simulink model "EV_thermal_charger_2015a_jmaab"  (R2015a)
settings: Solver=ode3  StartTime=0.0  StopTime=1800  FixedStep=sampling_time  RelTol=1e-3
PreLoadFcn:
  | run('init_setting.m')
PostLoadFcn:
  | %set_param(gcs, 'SimulationCommand', 'update');
  | %load('save_param/save_P_Charger', 'P_Charger');
  | %load('save_param/save_T_User_set_temp_degC','T_User_set_temp_degC');
  | %load('save_param/save_ENV_PNT_PTTH_Temp_add_degC','ENV_PNT_PTTH_Temp_add_degC');
  | %load('save_param/save_ENV_PNT_CABIN_Temp_add_degC','ENV_PNT_CABIN_Temp_add_degC');
  | %load('save_param/save_ENV_PNT_PHI_Sunlight_W','ENV_PNT_PHI_Sunlight_W');
  | %load('save_param/save_ENV_PNT_Outside_Temp_ini_degC','ENV_PNT_Outside_Temp_ini_degC');
undefined symbols (not defined in the file or in its folder): BK_PNT_Pow_UL, BK_PNT_ReGene_vel_limit_DN_kmph, BK_PNT_ReGene_vel_limit_UP_kmph, BK_PNT_Tau_brake, Brk_LL, Brk_PGain, Brk_UL, BT_PNT_Hi_C_pol_hi_batt, BT_PNT_Hi_Capa_hi_batt_F, BT_PNT_Hi_ocv_SOC_hi_batt_OCV_V_table, BT_PNT_Hi_ocv_SOC_hi_batt_OCV_V_table_x_SOC, BT_PNT_Hi_R_hi_batt_cell, BT_PNT_Hi_R_pol_hi_batt, BT_PNT_Hi_SOC_MAX_hi_batt, BT_PNT_Hi_SOC_MIN_hi_batt, BT_PNT_Hi_SOC_START_hi_batt, BT_PNT_Lo_Capa_lo_batt_F, BT_PNT_Lo_ocv_SOC_lo_batt_OCV_V_table, BT_PNT_Lo_ocv_SOC_lo_batt_OCV_V_table_x_SOC, BT_PNT_Lo_R_lo_batt_ohm, BT_PNT_Lo_SOC_MAX_lo_batt, BT_PNT_Lo_SOC_MIN_lo_batt, BT_PNT_Lo_SOC_START_lo_batt, BTTH_CNT_P_BT_Heater_W, BTTH_CNT_P_BT_Heater_W_x_BTCells_degC, BTTH_CNT_Voltage_BTFan_V, BTTH_CNT_Voltage_BTFan_V_x_BTCells_degC, BTTH_PNT_BT_Heat_Resi_KpW, BTTH_PNT_BT_Heat_Resi_KpW_x_Wind_m3ps, BTTH_PNT_BT_Heater2BTCells_Heat_Resi_KpW, BTTH_PNT_BT_Heater_Heat_Capa_JpK, BTTH_PNT_BTBlock2BTAir_Heat_Resi_KpW, BTTH_PNT_BTBlock_Heat_Capa_JpK, BTTH_PNT_BTCells2BTBlock_Heat_Resi_KpW, BTTH_PNT_BTCells_Heat_Capa_JpK, BTTH_PNT_v_BTFan_Wind_vel_mps, BTTH_PNT_v_BTFan_Wind_vel_mps_x_V_BTFan, CATH_CNT_P_Aircon_W_LL, CATH_CNT_P_Aircon_W_UL, CATH_CNT_P_Gain_Aircon, CATH_CNT_P_Gain_PTC_Heater, CATH_CNT_P_Gain_SeatHT, CATH_CNT_P_PTC_Heater, CATH_CNT_P_PTC_Heater_W_LL, CATH_CNT_P_PTC_Heater_W_UL, CATH_CNT_P_PTC_Heater_x_T_Outside_temp_degC, CATH_CNT_P_SeatHT_W_LL, CATH_CNT_P_SeatHT_W_UL, CATH_CNT_PGain_Temp_blowout, CATH_CNT_T_Aircon_Indoor_degC, CATH_CNT_T_Aircon_Indoor_degC_x_T_blowout_degC, CATH_CNT_T_PTC_Heater_degC_UL, CATH_CNT_T_SeatHT_Temp_degC, CATH_CNT_T_SeatHT_Temp_degC_x_T_blowout_degC, CATH_CNT_V_HVAC_Fan, CATH_CNT_V_HVAC_Fan_x_T_blowout_degC, CATH_CNT_V_RDFan_V, CATH_CNT_V_RDFan_x_P_Aircon_W, CATH_PNT_Air_Convection_Heat_Resi_KpW, CATH_PNT_Air_Convection_Heat_Resi_x_mps ... (+142)
undefined symbols (not defined in the file): ACC_D_Gain, ACC_I_Gain, ACC_P_Gain
libraries: METI_Lib_vehicle_model x52, simulink x35
(part 1 of 6)
PreSaveFcn:
  | %save('save_param/save_P_Charger', 'P_Charger');
  | %save('save_param/save_T_User_set_temp_degC', 'T_User_set_temp_degC');
  | %save('save_param/save_ENV_PNT_PTTH_Temp_add_degC', 'ENV_PNT_PTTH_Temp_add_degC');
  | %save('save_param/save_ENV_PNT_CABIN_Temp_add_degC', 'ENV_PNT_CABIN_Temp_add_degC');
  | %save('save_param/save_ENV_PNT_PHI_Sunlight_W', 'ENV_PNT_PHI_Sunlight_W');
  | %save('save_param/save_ENV_PNT_Outside_Temp_ini_degC', 'ENV_PNT_Outside_Temp_ini_degC');
settings Model: Creator=AZAPA  LastModifiedBy=E00026
settings OptimizationCC: EfficientMapNaN2IntZero=off
settings DebuggingCC: SFInvalidInputDataAccessInChartInitDiag=none  SFNoUnconditionalDefaultTransitionDiag=none
settings HardwareCC: TargetBitPerPointer=64  TargetLongLongMode=on  TargetIntDivRoundTo=Zero  TargetEndianess=LittleEndian  TargetWordSize=64  TargetHWDeviceType=MATLAB Host  ProdEqTarget=off
settings CodeAppCC: MaxIdLength=128
settings GRTTargetCC: CombineOutputUpdateFcns=off  GRTInterface=on

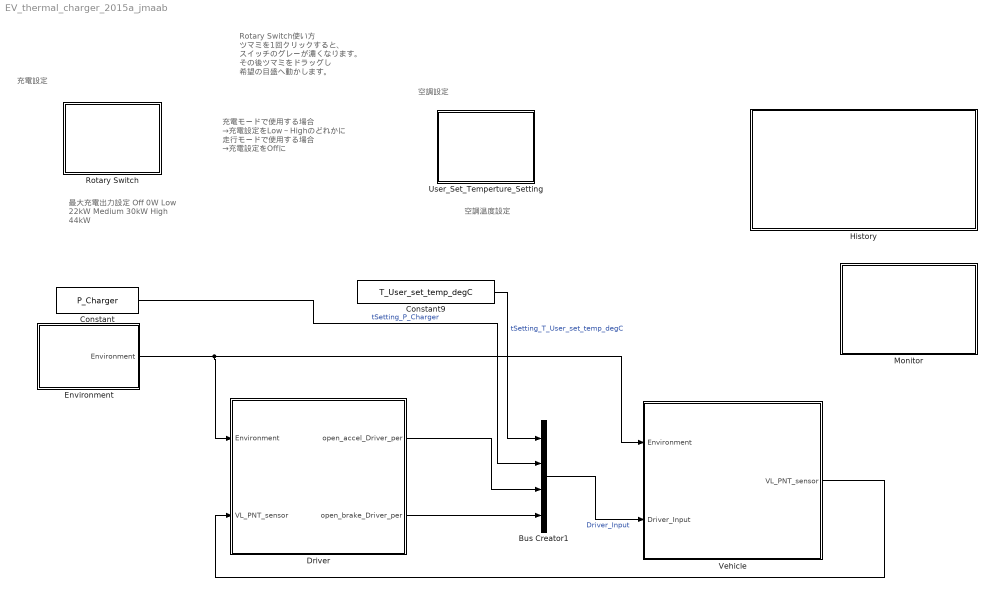
== system EV_thermal_charger_2015a_jmaab ==
  note: 充電モードで使用する場合
      | →充電設定をLow～Highのどれかに
      |
      | 走行モードで使用する場合
      | →充電設定をOffに
  note: 充電設定
  note: 空調温度設定
  note: 空調設定
  note: 最大充電出力設定
      | Off 0W
      | Low 22kW
      | Medium 30kW
      | High 44kW
  note: Rotary Switch使い方
      | ツマミを1回クリックすると、
      | スイッチのグレーが濃くなります。
      | その後ツマミをドラッグし
      | 希望の目盛へ動かします。
  Bus Creator1 : BusCreator  Inputs=4
  Constant : Constant  Value=P_Charger
  Constant9 : Constant  Value=T_User_set_temp_degC
  Driver : Subsystem
      mask Display: image(imread('picture\ドライバ.png'))
  Environment : Subsystem
  History : Subsystem
  Monitor : Subsystem
  Rotary Switch : Subsystem  DialogController=hmiCreateDDGDialog  IsWebBlock=on  mask(MathWorksWebBlock){webBlockId=88c50587-98df-4da6-abec-7a3537762cf8, webBlockType=discreteknob, ShowInLibBrowser=on, ShowInitialText=on, HMISrcModelName=tpeaf5fb4a_b3bf_4f70_b0c1_9b4aa428c6f5}
      mask prompts: webBlockId "WebBlock Id"; webBlockType "WebBlock Type"; HMISrcModelName "Source Model"
      mask help: 値を設定してパラメーターまたは変数を調整します。
      mask Help: helpview([docroot '/mapfiles/simulink.map'], 'hmi_rotary_switch')
      mask Display:
      | if strcmp(get_param(bdroot(gcb),'BlockDiagramType'),'library')
      |  image([(matlabroot) '/toolbox/simulink/hmi/icons/DiscreteKnob.png'])
      | end
  User_Set_Temperture_Setting : Subsystem  DialogController=hmiCreateDDGDialog  IsWebBlock=on  mask(MathWorksWebBlock){webBlockId=37ee7956-8de0-466d-b842-934e6700f2c4, webBlockType=discreteknob, ShowInLibBrowser=on, ShowInitialText=on, HMISrcModelName=tpeaf5fb4a_b3bf_4f70_b0c1_9b4aa428c6f5}
      mask prompts: webBlockId "WebBlock Id"; webBlockType "WebBlock Type"; HMISrcModelName "Source Model"
      mask help: 値を設定してパラメーターまたは変数を調整します。
      mask Help: helpview([docroot '/mapfiles/simulink.map'], 'hmi_rotary_switch')
      mask Display:
      | if strcmp(get_param(bdroot(gcb),'BlockDiagramType'),'library')
      |  image([(matlabroot) '/toolbox/simulink/hmi/icons/DiscreteKnob.png'])
      | end
  Vehicle : Subsystem
      mask Display: image(imread('picture\電気負荷.png'))
  wires:
  Vehicle/1(VL_PNT_sensor) -> Driver/2(VL_PNT_sensor)
  Driver/1(open_accel_Driver_per) -> Bus Creator1/3
  Driver/2(open_brake_Driver_per) -> Bus Creator1/4
  Constant/1 -> Bus Creator1/2  "tSetting_P_Charger"
  Constant9/1 -> Bus Creator1/1  "tSetting_T_User_set_temp_degC"
  Environment/1(Environment) -> Driver/1(Environment), Vehicle/1(Environment)
  Bus Creator1/1 -> Vehicle/2(Driver_Input)  "Driver_Input"

== system EV_thermal_charger_2015a_jmaab/Driver ==
  Environment : Inport
  VL_PNT_sensor : Inport  Port=2
  Bus Selector : BusSelector  OutputSignals=tgt_v_kmph
  Bus Selector1 : BusSelector  OutputSignals=v_VL_PNT_kmph
  Caliculate_Driving_State : Subsystem
  Caliculate_Opeining_Accel : Subsystem
  Caliculate_Opening_Brake : Subsystem
  Memory2 : Memory  InheritSampleTime=on
  open_accel_Driver_per : Outport
  open_brake_Driver_per : Outport  Port=2
  tag scope: tScope_accel=global, tScope_brake=global, tScope_v_Vehicle=global, tScope_v_tgt=global
  wires:
  Memory2/1 -> [tScope_v_Vehicle], Caliculate_Opening_Brake/1(v_VL_PNT_kmph), Caliculate_Opeining_Accel/1(v_VL_PNT_kmph)
  Caliculate_Opeining_Accel/1(open_accel_Driver_per) -> open_accel_Driver_per/1, [tScope_accel], Caliculate_Opening_Brake/3(open_accel_Driver_per)
  Caliculate_Opening_Brake/1(open_brake_Driver_per) -> open_brake_Driver_per/1, [tScope_brake], Caliculate_Driving_State/1(open_brake_Driver_per)
  VL_PNT_sensor/1 -> Bus Selector1/1
  Environment/1 -> Bus Selector/1
  Bus Selector/1 -> Caliculate_Driving_State/2(tgt_v_kmph), Caliculate_Opening_Brake/2(tgt_v_kmph), Caliculate_Opeining_Accel/2(tgt_v_kmph), [tScope_v_tgt]  "<tgt_v_kmph>"
  Bus Selector1/1 -> Memory2/1  "<v_VL_PNT_kmph>"

== system EV_thermal_charger_2015a_jmaab/Environment ==
  note: 車外気温設定
      | VeryCold -30℃
      | Cold 0℃
      | Warm 20℃
      | VeryHot 40℃
  note: 気象設定（直射日光の有無）
      | Night 日射熱量 0W
      | Cloudy 日射熱量 100W
      | Sunny 日射熱量 1000W
  note: 気象条件設定
  note: Rotary Switch使い方
      | ツマミを1回クリックすると、
      | スイッチのグレーが濃くなります。
      | その後ツマミをドラッグし
      | 希望の目盛へ動かします。
  note: スタート時
      | 車室温度設定
      | 直射日光下で駐車した状態では
      | 車室温度は外気温より高くなる
  note: スタート時パワトレ・パワエレ
      | HOT/COLD設定
      | COLD 外気温と同じ温度から
      | HOT 外気温+40℃から
  note: 車両条件設定
  note: 充電モードでは走行しないので
      | 目標車速を0にする
  Bus Creator2 : BusCreator  Inputs=5
  CABIN_Temp_add : Subsystem  DialogController=hmiCreateDDGDialog  IsWebBlock=on  mask(MathWorksWebBlock){webBlockId=d4d8367f-57c7-4656-8fe5-c97b2c29613b, webBlockType=discreteknob, ShowInLibBrowser=on, ShowInitialText=on, HMISrcModelName=tpeaf5fb4a_b3bf_4f70_b0c1_9b4aa428c6f5}
      mask prompts: webBlockId "WebBlock Id"; webBlockType "WebBlock Type"; HMISrcModelName "Source Model"
      mask help: 値を設定してパラメーターまたは変数を調整します。
      mask Help: helpview([docroot '/mapfiles/simulink.map'], 'hmi_rotary_switch')
      mask Display:
      | if strcmp(get_param(bdroot(gcb),'BlockDiagramType'),'library')
      |  image([(matlabroot) '/toolbox/simulink/hmi/icons/DiscreteKnob.png'])
      | end
  COLD/HOT : Subsystem  DialogController=hmiCreateDDGDialog  IsWebBlock=on  mask(MathWorksWebBlock){webBlockId=ec53c6ff-a8cf-4237-bb99-052eb2fa9088, webBlockType=discreteknob, ShowInLibBrowser=on, ShowInitialText=on, HMISrcModelName=tpeaf5fb4a_b3bf_4f70_b0c1_9b4aa428c6f5}
      mask prompts: webBlockId "WebBlock Id"; webBlockType "WebBlock Type"; HMISrcModelName "Source Model"
      mask help: 値を設定してパラメーターまたは変数を調整します。
      mask Help: helpview([docroot '/mapfiles/simulink.map'], 'hmi_rotary_switch')
      mask Display:
      | if strcmp(get_param(bdroot(gcb),'BlockDiagramType'),'library')
      |  image([(matlabroot) '/toolbox/simulink/hmi/icons/DiscreteKnob.png'])
      | end
  Constant3 : Constant  Value=P_Charger
  Constant4 : Constant  Value=0
  Constant5 : Constant  Value=ENV_PNT_PTTH_Temp_add_degC
  Constant6 : Constant  Value=ENV_PNT_CABIN_Temp_add_degC
  Constant7 : Constant  Value=ENV_PNT_PHI_Sunlight_W
  Constant8 : Constant  Value=ENV_PNT_Outside_Temp_ini_degC
  From Workspace : FromWorkspace  VariableName=jc08  SampleTime=0
  From Workspace2 : FromWorkspace  VariableName=wltc_class3b  SampleTime=0
  Manual Switch2 : ManualSwitch  CurrentSetting=0
  Outside_Temperture_Setting : Subsystem  DialogController=hmiCreateDDGDialog  IsWebBlock=on  mask(MathWorksWebBlock){webBlockId=d913990a-62c7-4b41-8bbd-c48c7457c0a7, webBlockType=discreteknob, ShowInLibBrowser=on, ShowInitialText=on, HMISrcModelName=tpeaf5fb4a_b3bf_4f70_b0c1_9b4aa428c6f5}
      mask prompts: webBlockId "WebBlock Id"; webBlockType "WebBlock Type"; HMISrcModelName "Source Model"
      mask help: 値を設定してパラメーターまたは変数を調整します。
      mask Help: helpview([docroot '/mapfiles/simulink.map'], 'hmi_rotary_switch')
      mask Display:
      | if strcmp(get_param(bdroot(gcb),'BlockDiagramType'),'library')
      |  image([(matlabroot) '/toolbox/simulink/hmi/icons/DiscreteKnob.png'])
      | end
  Sunlight_Heat_Flux_Setting : Subsystem  DialogController=hmiCreateDDGDialog  IsWebBlock=on  mask(MathWorksWebBlock){webBlockId=bc677613-1ce2-4713-9922-c87efda7b29b, webBlockType=discreteknob, ShowInLibBrowser=on, ShowInitialText=on, HMISrcModelName=tpeaf5fb4a_b3bf_4f70_b0c1_9b4aa428c6f5}
      mask prompts: webBlockId "WebBlock Id"; webBlockType "WebBlock Type"; HMISrcModelName "Source Model"
      mask help: 値を設定してパラメーターまたは変数を調整します。
      mask Help: helpview([docroot '/mapfiles/simulink.map'], 'hmi_rotary_switch')
      mask Display:
      | if strcmp(get_param(bdroot(gcb),'BlockDiagramType'),'library')
      |  image([(matlabroot) '/toolbox/simulink/hmi/icons/DiscreteKnob.png'])
      | end
  Switch : Switch  Criteria=u2 > Threshold
  Environment : Outport
  wires:
  Constant7/1 -> Bus Creator2/1  "PHI_Environment_Sunlight_W"
  Constant5/1 -> Bus Creator2/3  "add_T_Environment_PTTH_ELTH_degC"
  Constant6/1 -> Bus Creator2/4  "add_T_Environment_CATH_degC"
  Constant8/1 -> Bus Creator2/2  "ini_T_Environment_Outside_degC"
  Bus Creator2/1 -> Environment/1  "Environment"
  Constant3/1 -> Switch/2
  Constant4/1 -> Switch/1
  From Workspace2/1 -> Manual Switch2/2
  From Workspace/1 -> Manual Switch2/1
  Manual Switch2/1 -> Switch/3
  Switch/1 -> Bus Creator2/5  "tgt_v_kmph"

== system EV_thermal_charger_2015a_jmaab/History ==

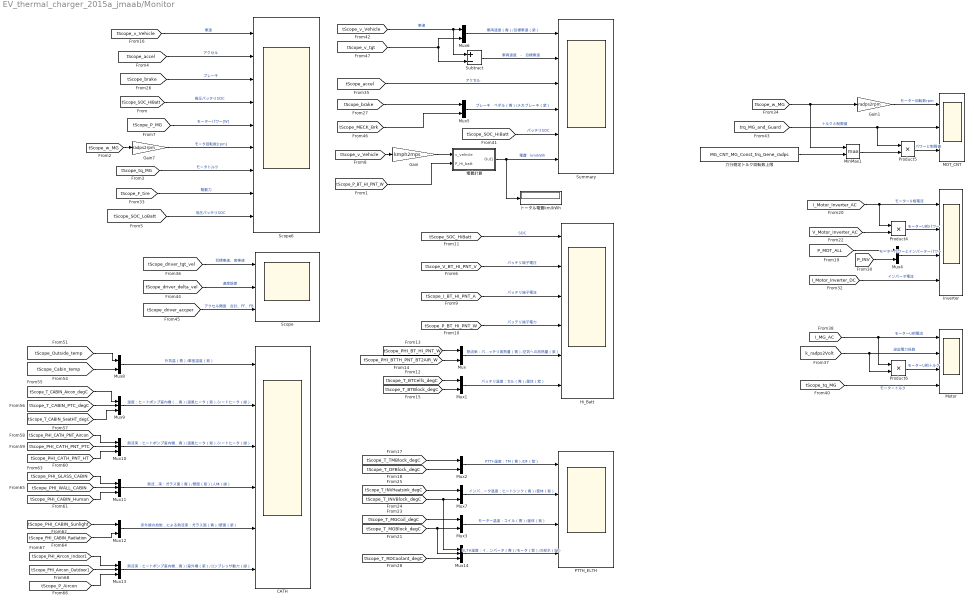
== system EV_thermal_charger_2015a_jmaab/Monitor ==
  CATH : Scope  NumInputPorts=6
      settings: TimeRange=auto  MaxDataPoints=5000  SaveToWorkspace=off  SaveName=ScopeData12  YMin=20~20~-35000~-0~0~-15000  YMax=70~70~5000~4500~1000~35000  SampleTime=-1  DataFormat=Array
  Gain : Gain  Gain=kmph2mps
  Gain1 : Gain  Gain=radps2rpm
  Gain7 : Gain  Gain=radps2rpm
  Hi_Batt : Scope  NumInputPorts=6
      settings: TimeRange=auto  MaxDataPoints=5000  SaveToWorkspace=off  SaveName=ScopeData4  YMin=44.5~337.5~-100~-40000~-100~20  YMax=50~352.5~125~40000~1000~20.4  SampleTime=-1  DataFormat=Array
  Inverter : Scope  NumInputPorts=4
      settings: TimeRange=1800  MaxDataPoints=5000  SaveToWorkspace=off  SaveName=ScopeData15  YMin=-30~-7500~-12500~-30  YMax=60~15000~22500~60  SampleTime=-1  DataFormat=Array
  MOT_CNT : Scope  NumInputPorts=3
      settings: TimeRange=1800  MaxDataPoints=5000  SaveToWorkspace=off  SaveName=ScopeData11  YMin=-500~-350~-125000  YMax=7000~350~125000  SampleTime=-1  DataFormat=Array
  MinMax1 : MinMax  Function=max  Inputs=2
  Motor : Scope  NumInputPorts=4
      settings: TimeRange=1800  MaxDataPoints=5000  SaveToWorkspace=off  SaveName=ScopeData14  YMin=-2.5~0.75~-5~-10  YMax=35~1.025~40~100  SampleTime=-1  DataFormat=Array
  Mux{,1..8,12} (10 alike) : Mux  Inputs=2
  Mux{9..11,13..14} (5 alike) : Mux  Inputs=3
  PTTH_ELTH : Scope  NumInputPorts=4
      settings: TimeRange=1800  MaxDataPoints=5000  SaveToWorkspace=off  SaveName=ScopeData10  YMin=40~40~40~40  YMax=41~41.75~42~42  SampleTime=-1  DataFormat=Array
  Product4 : Product
  Product5 : Product
  Product6 : Product
  Scope : Scope  NumInputPorts=3
      settings: TimeRange=1800  MaxDataPoints=5000  SaveToWorkspace=off  SaveName=ScopeData8  YMin=0~-0.4~-20  YMax=140~1.2~80  SampleTime=-1  DataFormat=Array
  Scope6 : Scope  NumInputPorts=9
      settings: TimeRange=186.7025  MaxDataPoints=5000  SaveToWorkspace=off  SaveName=ScopeData6  YMin=35~0~-1~45.37~-30000~2250~-100~-3000~74.175  YMax=55~50~1~45.48~30000~4000~100~2000~74.35  SampleTime=-1  DataFormat=Array
  Subtract : Sum  Inputs=+-
  Summary : Scope  NumInputPorts=6
      settings: TimeRange=auto  MaxDataPoints=5000  SaveToWorkspace=off  SaveName=ScopeData5  YMin=0~-0.6~0~0~41~0  YMax=150~0.1~70~5~50~9  SampleTime=-1  DataFormat=Array
  トータル電費km/kWh : Display
  力行側定トルク回転数上限 : Constant  Value=MG_CNT_MG_Const_trq_Gene_radps
  電費計算 : Subsystem
  wires:
  [tScope_v_Vehicle] -> Scope6/1  "車速"
  [tScope_accel] -> Scope6/2  "アクセル"
  [tScope_brake] -> Scope6/3  "ブレーキ"
  [tScope_SOC_HiBatt] -> Scope6/4  "高圧バッテリSOC"
  Gain7/1 -> Scope6/6  "モータ回転数[rpm]"
  [tScope_tq_MG] -> Scope6/7  "モータトルク"
  [tScope_F_tire] -> Scope6/8  "駆動力"
  Mux4/1 -> Inverter/3  "モーターパワーとインバーターパワー"
  [I_Motor_Inverter_AC] -> Product4/1, Inverter/1  "モーターU相電流"
  Product4/1 -> Inverter/2  "モーターU相パワー"
  [V_Motor_Inverter_AC] -> Product4/2
  [P_MOT_ALL] -> Mux4/1
  [P_INV] -> Mux4/2
  [I_Motor_Inverter_DC] -> Inverter/4  "インバータ電流"
  [trq_MG_and_Guard] -> Product5/1, MOT_CNT/2  "トルクと制限値"
  Product5/1 -> MOT_CNT/3  "パワーと制限値"
  力行側定トルク回転数上限/1 -> MinMax1/2
  MinMax1/1 -> Product5/2
  Gain1/1 -> MOT_CNT/1  "モーター回転数rpm"
  [tScope_w_MG] -> MinMax1/1, Gain1/1
  [I_MG_AC] -> Product6/1, Motor/1  "モーターU相電流"
  [k_radps2Volt] -> Product6/2, Motor/2  "逆起電力係数"
  Product6/1 -> Motor/3  "モーターU相トルク"
  [tScope_tq_MG] -> Motor/4  "モータートルク"
  Mux5/1 -> Summary/4  "ブレーキ　ペダル（青）/メカブレーキ（紫）"
  [tScope_MECK_Brk] -> Mux5/2
  [tScope_v_Vehicle] -> Subtract/1, Mux6/1  "車速"
  Mux6/1 -> Summary/1  "車両速度（青）/目標車速（紫）"
  Subtract/1 -> Summary/2  "車両速度　-　目標車速"
  [tScope_SOC_HiBatt] -> Summary/5  "バッテリSOC"
  [tScope_v_tgt] -> Mux6/2, Subtract/2
  [tScope_accel] -> Summary/3  "アクセル"
  [tScope_brake] -> Mux5/1
  [tScope_w_MG] -> Gain7/1
  [tScope_driver_tgt_vel] -> Scope/1  "目標車速、実車速"
  [tScope_driver_delta_vel] -> Scope/2  "速度誤差"
  [tScope_driver_accper] -> Scope/3  "アクセル開度　合計、FF、FB"
  電費計算/1(Out1) -> トータル電費km/kWh/1, Summary/6  "電費　km/kWh"
  [tScope_Outside_temp] -> Mux8/1
  [tScope_Cabin_temp] -> Mux8/2
  Mux8/1 -> CATH/1  "外気温（青）/車室温度（紫）"
  Mux9/1 -> CATH/2  "温度：ヒートポンプ室内機（青）/温風ヒータ（紫）/シートヒータ（緑）"
  [tScope_T_CABIN_Aicon_degC] -> Mux9/1
  [tScope_T_CABIN_PTC_degC] -> Mux9/2
  [tScope_T_CABIN_SeatHT_degC] -> Mux9/3
  Mux10/1 -> CATH/3  "熱流束：ヒートポンプ室内機（青）/温風ヒータ（紫）/シートヒータ（緑）"
  [tScope_PHI_CATH_PNT_Aircon] -> Mux10/1
  [tScope_PHI_CATH_PNT_PTC] -> Mux10/2
  [tScope_PHI_CATH_PNT_HT] -> Mux10/3
  Mux11/1 -> CATH/4  "熱流束：ガラス面（青）/壁面（紫）/人体（緑）"
  Mux12/1 -> CATH/5  "赤外線の放射による熱流束：ガラス面（青）/壁面（紫）"
  [tScope_PHI_CABIN_Sunlight] -> Mux12/1
  [tScope_PHI_CABIN_Radiation] -> Mux12/2
  [tScope_PHI_WALL_CABIN] -> Mux11/2
  [tScope_PHI_GLASS_CABIN] -> Mux11/1
  [tScope_PHI_CABIN_Human] -> Mux11/3
  Mux13/1 -> CATH/6  "熱流束：ヒートポンプ室内機（青）/室外機（紫）/コンプレッサ動力（緑）"
  [tScope_PHI_Aircon_Outdoor1] -> Mux13/2
  [tScope_PHI_Aircon_Indoor1] -> Mux13/1
  [tScope_P_Aircon] -> Mux13/3
  [tScope_v_Vehicle] -> Gain/1
  [tScope_P_BT_HI_PNT_W] -> 電費計算/2(P_Hi_batt)
  [tScope_SOC_LoBatt] -> Scope6/9  "低圧バッテリSOC"
  [tScope_P_MG] -> Scope6/5  "モーターパワー[W]"
  [tScope_SOC_HiBatt] -> Hi_Batt/1  "SOC"
  [tScope_V_BT_HI_PNT_V] -> Hi_Batt/2  "バッテリ端子電圧"
  [tScope_I_BT_HI_PNT_A] -> Hi_Batt/3  "バッテリ端子電流"
  Mux1/1 -> Hi_Batt/6  "バッテリ温度：セル（青）/筐体（紫）"
  Mux/1 -> Hi_Batt/5  "熱流束：バッテリ発熱量（青）/空気への放熱量（紫）"
  [tScope_P_BT_HI_PNT_W] -> Hi_Batt/4  "バッテリ端子電力"
  [tScope_PHI_BT_HI_PNT_W] -> Mux/1
  [tScope_PHI_BTTH_PNT_BT2AIR_W] -> Mux/2
  [tScope_T_BTCells_degC] -> Mux1/1
  [tScope_T_BTBlock_degC] -> Mux1/2
  Gain/1 -> 電費計算/1(v_vehicle)
  [tScope_T_DFBlock_degC] -> Mux2/2
  [tScope_T_TMBlock_degC] -> Mux2/1
  [tScope_T_MGCoil_degC] -> Mux3/1
  [tScope_T_MGBlock_degC] -> Mux14/2, Mux3/2
  [tScope_T_INVHeatsink_degC] -> Mux7/1
  [tScope_T_INVBlock_degC] -> Mux14/1, Mux7/2
  [tScope_T_RDCoolant_degC] -> Mux14/3
  Mux2/1 -> PTTH_ELTH/1  "PTTH温度：TM（青）/DF（紫）"
  Mux7/1 -> PTTH_ELTH/2  "インバータ温度：ヒートシンク（青）/筐体（紫）"
  Mux3/1 -> PTTH_ELTH/3  "モーター温度：コイル（青）/筐体（紫）"
  Mux14/1 -> PTTH_ELTH/4  "ELTH温度：インバータ（青）/モータ（紫）/冷却水（緑）"

== system EV_thermal_charger_2015a_jmaab/Rotary Switch ==

== system EV_thermal_charger_2015a_jmaab/User_Set_Temperture_Setting ==

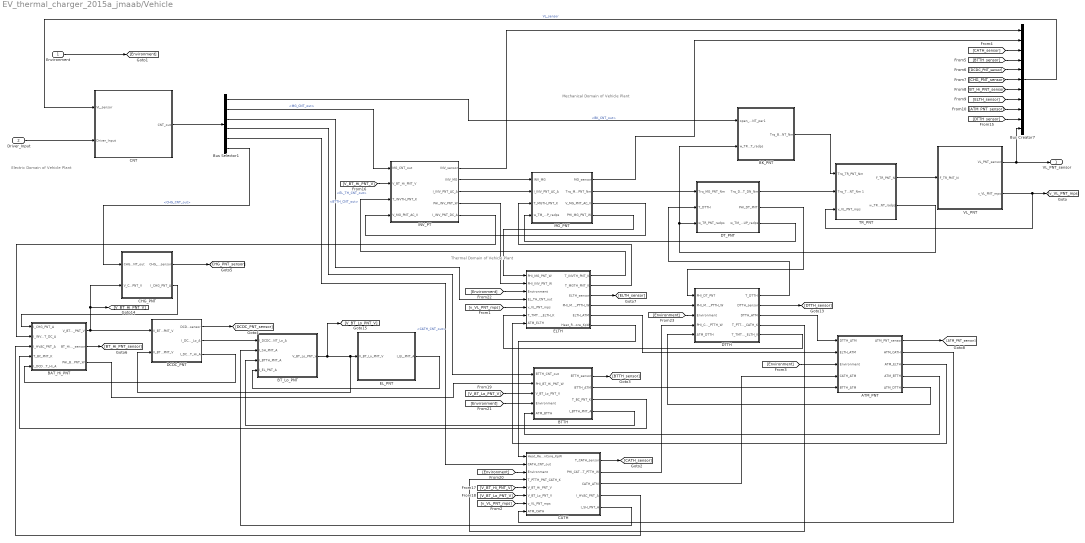
== system EV_thermal_charger_2015a_jmaab/Vehicle ==
  note: Thermal Domain of Vehicle Plant
  note: Electric Domain
      |  of Vehicle Plant
  note: Mechanical Domain of Vehicle Plant
  Environment : Inport
  Driver_Input : Inport  Port=2
  ATM_PNT : Subsystem
  BAT_Hi_PNT : Subsystem
      mask Display: image(imread('Li-INOバッテリ.png'))
  BK_PNT : Subsystem
      mask Display: image(imread('picture\ブレーキ02.png'))
  BTTH : Subsystem
      mask Display: image(imread('Li-INOバッテリ.png'))
  BT_Lo_PNT : Subsystem
      mask Display: image(imread('picture\バッテリー.png'))
  Bus Creator7 : BusCreator  Inputs=11
  Bus Selector1 : BusSelector  OutputSignals=BK_CNT_out,MG_CNT_out,EL_TH_CNT_out,BTTH_CNT_out,CATH_CNT_out,CHG_CNT_out
  CATH : Subsystem
      mask Display: image(imread('熱マネ　カーエアコン.jpg'))
  CHG_PNT : Subsystem
      mask Display: image(imread('電気　有線充電器.jpg'))
  CNT : Subsystem
      mask Display: image(imread('ECU.png'))
  DCDC_PNT : Subsystem
      mask Display: image(imread('電気　降圧DCDCコンバータ.jpg'))
  DTTH : Subsystem
      mask Display: image(imread('パワトレ　AT.jpg'))
  DT_PNT : Subsystem
      mask Display: image(imread('パワトレ　AT.jpg'))
  ELTH : Subsystem
      mask Display: image(imread('picture\インバーター01.png'))
  EL_PNT : Subsystem
      mask Display: image(imread('picture\電気負荷.png'))
  INV_PT : Subsystem
      mask Display: image(imread('picture\インバーター01.png'))
  MG_PNT : Subsystem
      mask Display: image(imread('picture\モータドライブシステム03.png'))
  TR_PNT : Subsystem
      mask Display: image(imread('picture\タイヤ01.png'))
  VL_PNT : Subsystem
      mask Display: image(imread('自動車　EV車両.jpg'))
  VL_PNT_sensor : Outport
  wires:
  TR_PNT/2(ｗ_TR_PNT_radps) -> BK_PNT/2("w_TR_PNT_radps "), DT_PNT/3(w_TR_PNT_radps)
  BK_PNT/1(Trq_BK_PNT_Nm) -> TR_PNT/1("Trq_TR_PNT_Nm ")
  VL_PNT/2(v_VL_PNT_mps) -> TR_PNT/3(v_VL_PNT_mps), [v_VL_PNT_mps]
  TR_PNT/1("F_TR_PNT_N ") -> VL_PNT/1(F_TR_PNT_N)
  VL_PNT/1(VL_PNT_sensor) -> VL_PNT_sensor/1, Bus Creator7/11
  BTTH/1(BTTH_sensor) -> [BTTH_sensor]
  Environment/1 -> [Environment]
  DT_PNT/1(Trq_DF_PNT_DN_Nm) -> TR_PNT/2(Trq_TR_PNT_Nm 1)
  CNT/1(CNT_out) -> Bus Selector1/1
  Driver_Input/1 -> CNT/2(Driver_Input)
  Bus Creator7/1 -> CNT/1(VL_sensor)  "VL_sensor"
  INV_PT/1(INV_sensor) -> Bus Creator7/1
  DT_PNT/3(w_TM_PNT_UP_radps) -> MG_PNT/4(w_TM_PNT_UP_radps)
  INV_PT/2(INV_MG) -> MG_PNT/1(INV_MG)
  INV_PT/3(I_INV_PNT_AC_A) -> MG_PNT/2(I_INV_PNT_AC_A)
  MG_PNT/1(MG_sensor) -> Bus Creator7/2
  MG_PNT/2(Trq_MG_PNT_Nm) -> DT_PNT/1(Trq_MG_PNT_Nm)
  MG_PNT/3(V_MG_PNT_AC_V) -> INV_PT/4(V_MG_PNT_AC_V)
  CATH/1(T_CATH_sensor) -> [CATH_sensor]
  [v_VL_PNT_mps] -> CATH/7(v_VL_PNT_mps)
  BAT_Hi_PNT/1(V_BT_Hi_PNT_V) -> DCDC_PNT/1(V_BT_Hi_PNT_V), [V_BT_Hi_PNT_V], CHG_PNT/2(V_CHG_PNT_V)
  INV_PT/5(I_INV_PNT_DC_A) -> BAT_Hi_PNT/2(I_INV_PNT_DC_A)
  CATH/4(I_HVAC_PNT_A) -> BAT_Hi_PNT/3(I_HVAC_PNT_A)
  BTTH/3(T_BC_PNT_K) -> BAT_Hi_PNT/4(T_BC_PNT_K)
  BAT_Hi_PNT/2(BT_Hi_PNT_sensor) -> [BT_Hi_PNT_sensor]
  BAT_Hi_PNT/3(PHI_BT_Hi_PNT_W) -> BTTH/2(PHI_BT_Hi_PNT_W)
  BT_Lo_PNT/1(V_BT_Lo_PNT_V) -> DCDC_PNT/2(V_BT_Lo_PNT_V), EL_PNT/1(V_BT_Lo_PNT_V), [V_BT_Lo_PNT_V]
  CATH/5(I_SH_PNT_A) -> BT_Lo_PNT/2(I_SH_PNT_A)
  BTTH/4(I_BTTH_PNT_A) -> BT_Lo_PNT/3(I_BTTH_PNT_A)
  EL_PNT/1(I_EL_PNT_A) -> BT_Lo_PNT/4(I_EL_PNT_A)
  INV_PT/4(PHI_INV_PNT_W) -> ELTH/2(PHI_INV_PNT_W)
  MG_PNT/4(PHI_MG_PNT_W) -> ELTH/1(PHI_MG_PNT_W)
  [v_VL_PNT_mps] -> ELTH/5(v_VL_PNT_mps)
  ELTH/1(T_INVTH_PNT_K) -> INV_PT/3(T_INVTH_PNT_K)
  ELTH/2(T_MGTH_PNT_K) -> MG_PNT/3(T_MGTH_PNT_K)
  ELTH/6(Heat_Resi_ELTH_PNT_AirconCore_KpW) -> CATH/1(Heat_Resi_ELTH_PNT_AirconCore_KpW)
  ELTH/3(ELTH_sensor) -> [ELTH_sensor]
  Bus Selector1/1 -> BK_PNT/1(open_brake_BK_CNT_per1)  "<BK_CNT_out>"
  Bus Selector1/2 -> INV_PT/1(MG_CNT_out)  "<MG_CNT_out>"
  Bus Selector1/3 -> ELTH/4(EL_TH_CNT_out)  "<EL_TH_CNT_out>"
  Bus Selector1/4 -> BTTH/1(BTTH_CNT_out)  "<BTTH_CNT_out>"
  Bus Selector1/6 -> CHG_PNT/1(CHG_CNT_out)  "<CHG_CNT_out>"
  Bus Selector1/5 -> CATH/2(CATH_CNT_out)  "<CATH_CNT_out>"
  ATM_PNT/2(ATM_CATH) -> CATH/8(ATM_CATH)
  CATH/3(CATH_ATM) -> ATM_PNT/4(CATH_ATM)
  CHG_PNT/2(I_CHG_PNT_A) -> BAT_Hi_PNT/1(I_CHG_PNT_A)
  CHG_PNT/1(CHG_PNT_sensor) -> [CHG_PNT_sensor]
  DCDC_PNT/3(I_DCDC_PNT_Hi_A) -> BAT_Hi_PNT/5(I_DCDC_PNT_Hi_A)
  DCDC_PNT/1(DCDC_PNT_sensor) -> [DCDC_PNT_sensor]
  DCDC_PNT/2(I_DCDC_PNT_Lo_A) -> BT_Lo_PNT/1(I_DCDC_PNT_Lo_A)
  ATM_PNT/3(ATM_ELTH) -> ELTH/7(ATM_ELTH)
  ELTH/4(PHI_MGTH_PNT_PTTH_W) -> DTTH/2(PHI_MGTH_PNT_PTTH_W)
  CATH/2(PHI_CATH_PNT_PTTH_W) -> DTTH/4(PHI_CATH_PNT_PTTH_W)
  ATM_PNT/5(ATM_DTTH) -> DTTH/5(ATM_DTTH)
  DTTH/5(T_TMTH_PNT_ELTH_K) -> ELTH/6(T_TMTH_PNT_ELTH_K)
  DTTH/2(DTTH_sensor) -> [DTTH_sensor]
  DTTH/4(T_PTTH_PNT_CATH_K) -> CATH/4(T_PTTH_PNT_CATH_K)
  DT_PNT/2(PHI_DT_PNT) -> DTTH/1(PHI_DT_PNT)
  DTTH/1(T_DTTH) -> DT_PNT/2(T_DTTH)
  ELTH/5(ELTH_ATM) -> ATM_PNT/2(ELTH_ATM)
  BTTH/2(BTTH_ATM) -> ATM_PNT/5(BTTH_ATM)
  ATM_PNT/1(ATM_PNT_sensor) -> [ATM_PNT_sensor]
  ATM_PNT/4(ATM_BTTH) -> BTTH/5(ATM_BTTH)
  [V_BT_Hi_PNT_V] -> INV_PT/2(V_BT_Hi_PNT_V)
  [V_BT_Hi_PNT_V] -> CATH/5(V_BT_Hi_PNT_V)
  [V_BT_Lo_PNT_V] -> CATH/6(V_BT_Lo_PNT_V)
  [V_BT_Lo_PNT_V] -> BTTH/3(V_BT_Lo_PNT_V)
  DTTH/3(DTTH_ATM) -> ATM_PNT/1(DTTH_ATM)
  [CATH_sensor] -> Bus Creator7/3
  [BTTH_sensor] -> Bus Creator7/4
  [DCDC_PNT_sensor] -> Bus Creator7/5
  [CHG_PNT_sensor] -> Bus Creator7/6
  [BT_Hi_PNT_sensor] -> Bus Creator7/7
  [ELTH_sensor] -> Bus Creator7/8
  [ATM_PNT_sensor] -> Bus Creator7/9
  [DTTH_sensor] -> Bus Creator7/10
  [Environment] -> ATM_PNT/3(Environment)
  [Environment] -> CATH/3(Environment)
  [Environment] -> BTTH/4(Environment)
  [Environment] -> ELTH/3(Environment)
  [Environment] -> DTTH/3(Environment)

== system EV_thermal_charger_2015a_jmaab/Driver/Caliculate_Driving_State ==
  open_brake_Driver_per : Inport
  tgt_v_kmph : Inport  Port=2
  Constant : Constant  Value=Thresh_Stop_vCar
  Constant4 : Constant  Value=0.1*sampling_time
  Constant6 : Constant  Value=-0.1*sampling_time
  Memory : Memory
  Relational Operator : RelationalOperator  Operator=>  OutDataTypeStr=boolean
  Relational Operator1 : RelationalOperator  Operator=<  OutDataTypeStr=boolean
  Relational Operator2 : RelationalOperator  Operator=<  OutDataTypeStr=boolean
  Sum : Sum  Inputs=|+-
  Switch{,1..3} (4 alike) : Switch  Criteria=u2 > Threshold  Threshold=0.5
  Terminator : Terminator
  停止 : Constant  Value=drivmode_STOP
  加速 : Constant  Value=drivmode_ACC
  定常1 : Constant  Value=drivmode_CONST
  減速力行 : Constant  Value=drivmode_GensokuRikko
  減速回生 : Constant  Value=drivmode_GensokuKaisei
  wires:
  Switch/1 -> Terminator/1  "state_driving"
  tgt_v_kmph/1 -> Relational Operator/1, Memory/1, Sum/1
  Relational Operator1/1 -> Switch1/2
  Constant4/1 -> Relational Operator1/2
  Relational Operator/1 -> Switch/2
  Constant/1 -> Relational Operator/2
  停止/1 -> Switch/3
  Sum/1 -> Relational Operator1/1, Relational Operator2/1
  減速回生/1 -> Switch2/1
  Switch3/1 -> Switch1/1
  Constant6/1 -> Relational Operator2/2
  Memory/1 -> Sum/2
  open_brake_Driver_per/1 -> Switch2/2
  減速力行/1 -> Switch2/3
  Relational Operator2/1 -> Switch3/2
  Switch2/1 -> Switch3/1
  定常1/1 -> Switch3/3
  加速/1 -> Switch1/3
  Switch1/1 -> Switch/1

== system EV_thermal_charger_2015a_jmaab/Driver/Caliculate_Opeining_Accel ==
  v_VL_PNT_kmph : Inport
  tgt_v_kmph : Inport  Port=2
  Constant : Constant  Value=VEHICLE_CNT_ACCper_UL
  Constant1 : Constant  Value=VEHICLE_CNT_ACCper_LL
  FB : Subsystem  mask{P_Gain=ACC_P_Gain, D_Gain=ACC_D_Gain, I_Gain=ACC_I_Gain}
      mask prompts: P_Gain "Pゲイン値"; D_Gain "Dゲイン値"; I_Gain "Iゲイン値"
  FF1 : Subsystem
  Mux : Mux  Inputs=2
  Mux1 : Mux  Inputs=3
  Saturation Dynamic : simulink/Discontinuities/Saturation Dynamic  OutMin=[]  OutMax=[]  OutDataTypeStr=Inherit: Same as second input  OutDataType=fixdt(1, 16)  OutScaling=2^-10  DoSatur=off
  Sum1 : Sum  Inputs=|-+
  Sum3 : Sum  Inputs=++|
  stopmode_calc : Subsystem
  open_accel_Driver_per : Outport
  tag scope: tScope_driver_accper=global, tScope_driver_delta_vel=global, tScope_driver_tgt_vel=global
  wires:
  Sum1/1 -> [tScope_driver_delta_vel], FB/1(delta_v_VL_kmph)
  v_VL_PNT_kmph/1 -> Mux/1, FF1/2(v_cal), Sum1/1
  Sum3/1 -> stopmode_calc/1(FF_FB_acc_per), Mux1/1
  FB/1(FB_open_accel_per) -> Sum3/1, Mux1/3
  FF1/1(per_acc_FF) -> Mux1/2, Sum3/2
  tgt_v_kmph/1 -> stopmode_calc/2(target_v_VL_kmph), FF1/1(v_tgt), Sum1/2, Mux/2
  Saturation Dynamic/1 -> open_accel_Driver_per/1  "open_accel_Driver_per"
  Mux/1 -> [tScope_driver_tgt_vel]  "目標車速 実車速"
  Mux1/1 -> [tScope_driver_accper]
  Constant/1 -> Saturation Dynamic/1
  Constant1/1 -> Saturation Dynamic/3
  stopmode_calc/1(open_accel_per) -> Saturation Dynamic/2

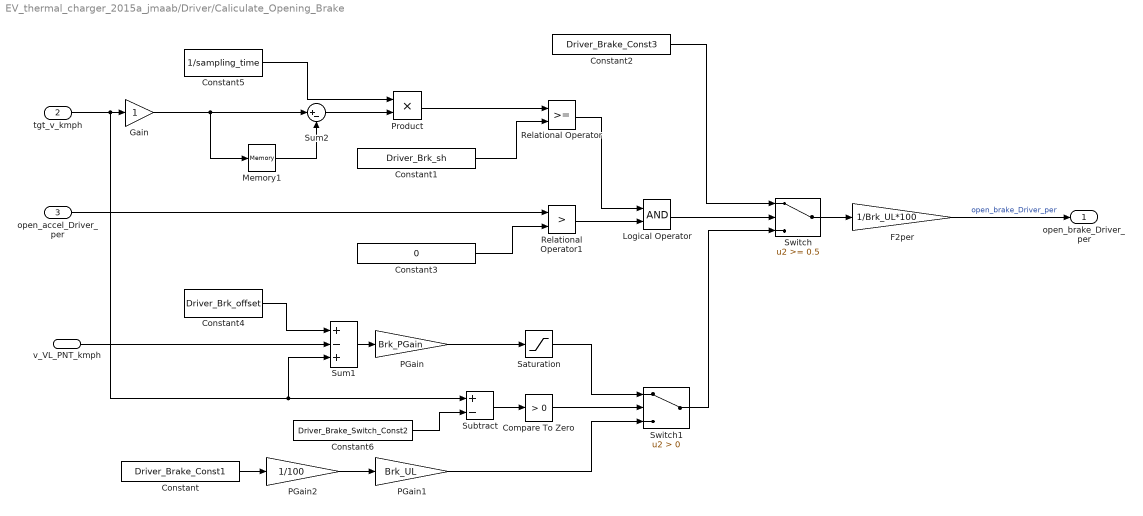
== system EV_thermal_charger_2015a_jmaab/Driver/Caliculate_Opening_Brake ==
  v_VL_PNT_kmph : Inport
  tgt_v_kmph : Inport  Port=2
  open_accel_Driver_per : Inport  Port=3
  Compare To Zero : simulink/Logic and Bit Operations/Compare To Zero  relop=>  OutDataTypeStr=boolean
  Constant : Constant  Value=Driver_Brake_Const1
  Constant1 : Constant  Value=Driver_Brk_sh
  Constant2 : Constant  Value=Driver_Brake_Const3
  Constant3 : Constant  Value=0
  Constant4 : Constant  Value=Driver_Brk_offset
  Constant5 : Constant  Value=1/sampling_time
  Constant6 : Constant  Value=Driver_Brake_Switch_Const2
  F2per : Gain  Gain=1/Brk_UL*100
  Gain : Gain
  Logical Operator : Logic  AllPortsSameDT=off  OutDataTypeStr=boolean
  Memory1 : Memory
  PGain : Gain  Gain=Brk_PGain
  PGain1 : Gain  Gain=Brk_UL
  PGain2 : Gain  Gain=1/100
  Product : Product
  Relational Operator : RelationalOperator  OutDataTypeStr=boolean
  Relational Operator1 : RelationalOperator  Operator=>  OutDataTypeStr=boolean
  Saturation : Saturate  UpperLimit=Brk_UL  LowerLimit=Brk_LL
  Subtract : Sum  Inputs=+-
  Sum1 : Sum  Inputs=+-+
  Sum2 : Sum  Inputs=|+-
  Switch : Switch  Threshold=0.5
  Switch1 : Switch  Criteria=u2 > Threshold
  open_brake_Driver_per : Outport
  wires:
  tgt_v_kmph/1 -> Gain/1, Subtract/1, Sum1/3
  Sum1/1 -> PGain/1
  PGain/1 -> Saturation/1
  Constant/1 -> PGain2/1
  PGain1/1 -> Switch1/3
  open_accel_Driver_per/1 -> Relational Operator1/1
  Memory1/1 -> Sum2/2
  Switch/1 -> F2per/1
  Product/1 -> Relational Operator/1
  Saturation/1 -> Switch1/1
  Switch1/1 -> Switch/3
  Constant2/1 -> Switch/1
  Constant1/1 -> Relational Operator/2
  Constant3/1 -> Relational Operator1/2
  Relational Operator/1 -> Logical Operator/1
  Relational Operator1/1 -> Logical Operator/2
  F2per/1 -> open_brake_Driver_per/1  "open_brake_Driver_per"
  v_VL_PNT_kmph/1 -> Sum1/2
  Constant4/1 -> Sum1/1
  Sum2/1 -> Product/2
  Constant5/1 -> Product/1
  Constant6/1 -> Subtract/2
  Subtract/1 -> Compare To Zero/1
  Compare To Zero/1 -> Switch1/2
  Logical Operator/1 -> Switch/2
  PGain2/1 -> PGain1/1
  Gain/1 -> Memory1/1, Sum2/1

== system EV_thermal_charger_2015a_jmaab/Environment/CABIN_Temp_add ==

== system EV_thermal_charger_2015a_jmaab/Environment/COLD//HOT ==

== system EV_thermal_charger_2015a_jmaab/Environment/Outside_Temperture_Setting ==

== system EV_thermal_charger_2015a_jmaab/Environment/Sunlight_Heat_Flux_Setting ==

== system EV_thermal_charger_2015a_jmaab/Monitor/電費計算 ==
  note: km
  note: m
  note: m/s
  note: W
  note: kWh
  note: kWsec
  note: Wsec
  v_vehicle : Inport
  P_Hi_batt : Inport  Port=2
  Constant : Constant  Value=0
  Divide_0wari : METI_Lib_vehicle_model/Divide_0wari
  Gain1 : Gain  Gain=1/1000
  Gain2 : Gain  Gain=1/3600
  Gain7 : Gain  Gain=1/1000
  Integrator : Integrator
  Integrator1 : Integrator
  Saturation Dynamic : simulink/Discontinuities/Saturation Dynamic  OutMin=[]  OutMax=[]  OutDataTypeStr=Inherit: Same as second input  OutDataType=fixdt(1, 16)  OutScaling=2^-10  DoSatur=off
  燃費表示上の上限値 : Constant  Value=50
  Out1 : Outport
  wires:
  Gain7/1 -> Divide_0wari/1
  燃費表示上の上限値/1 -> Saturation Dynamic/1
  Saturation Dynamic/1 -> Out1/1
  Divide_0wari/1 -> Saturation Dynamic/2
  Constant/1 -> Saturation Dynamic/3
  v_vehicle/1 -> Integrator/1
  Integrator/1 -> Gain7/1
  Gain2/1 -> Divide_0wari/2
  P_Hi_batt/1 -> Integrator1/1
  Integrator1/1 -> Gain1/1
  Gain1/1 -> Gain2/1

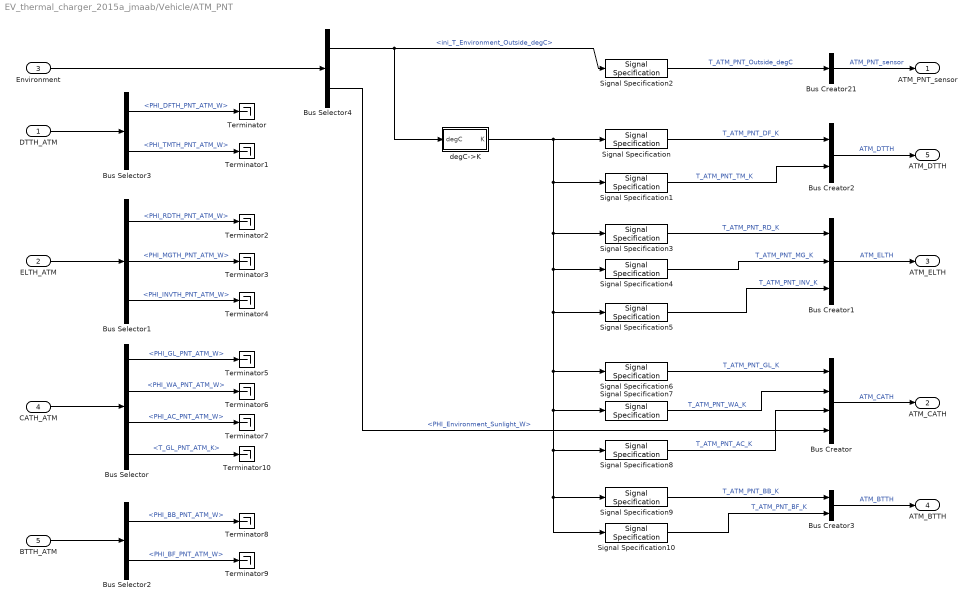
== system EV_thermal_charger_2015a_jmaab/Vehicle/ATM_PNT ==
  DTTH_ATM : Inport
  ELTH_ATM : Inport  Port=2
  Environment : Inport  Port=3
  CATH_ATM : Inport  Port=4
  BTTH_ATM : Inport  Port=5
  Bus Creator : BusCreator  Inputs=4
  Bus Creator1 : BusCreator  Inputs=3
  Bus Creator2 : BusCreator  Inputs=2
  Bus Creator21 : BusCreator  Inputs=1
  Bus Creator3 : BusCreator  Inputs=2
  Bus Selector : BusSelector  OutputSignals=PHI_GL_PNT_ATM_W,PHI_WA_PNT_ATM_W,PHI_AC_PNT_ATM_W,T_GL_PNT_ATM_K
  Bus Selector1 : BusSelector  OutputSignals=PHI_RDTH_PNT_ATM_W,PHI_MGTH_PNT_ATM_W,PHI_INVTH_PNT_ATM_W
  Bus Selector2 : BusSelector  OutputSignals=PHI_BB_PNT_ATM_W,PHI_BF_PNT_ATM_W
  Bus Selector3 : BusSelector  OutputSignals=PHI_DFTH_PNT_ATM_W,PHI_TMTH_PNT_ATM_W
  Bus Selector4 : BusSelector  OutputSignals=ini_T_Environment_Outside_degC,PHI_Environment_Sunlight_W
  Signal Specification{,1..10} (11 alike) : SignalSpecification
  Terminator{,1..10} (11 alike) : Terminator
  degC->K : Subsystem
  ATM_PNT_sensor : Outport
  ATM_CATH : Outport  Port=2
  ATM_ELTH : Outport  Port=3
  ATM_BTTH : Outport  Port=4
  ATM_DTTH : Outport  Port=5
  wires:
  degC->K/1(K) -> Signal Specification/1, Signal Specification3/1, Signal Specification6/1, Signal Specification10/1, Signal Specification9/1, Signal Specification8/1, Signal Specification7/1, Signal Specification5/1, Signal Specification4/1, Signal Specification1/1
  Signal Specification/1 -> Bus Creator2/1  "T_ATM_PNT_DF_K"
  Signal Specification1/1 -> Bus Creator2/2  "T_ATM_PNT_TM_K"
  Signal Specification3/1 -> Bus Creator1/1  "T_ATM_PNT_RD_K"
  Signal Specification4/1 -> Bus Creator1/2  "T_ATM_PNT_MG_K"
  Signal Specification5/1 -> Bus Creator1/3  "T_ATM_PNT_INV_K"
  Signal Specification6/1 -> Bus Creator/1  "T_ATM_PNT_GL_K"
  Signal Specification7/1 -> Bus Creator/2  "T_ATM_PNT_WA_K"
  Signal Specification8/1 -> Bus Creator/3  "T_ATM_PNT_AC_K"
  Signal Specification9/1 -> Bus Creator3/1  "T_ATM_PNT_BB_K"
  Signal Specification10/1 -> Bus Creator3/2  "T_ATM_PNT_BF_K"
  Bus Creator/1 -> ATM_CATH/1  "ATM_CATH"
  CATH_ATM/1 -> Bus Selector/1
  Bus Selector/1 -> Terminator5/1  "<PHI_GL_PNT_ATM_W>"
  Bus Selector/2 -> Terminator6/1  "<PHI_WA_PNT_ATM_W>"
  Bus Selector/3 -> Terminator7/1  "<PHI_AC_PNT_ATM_W>"
  Bus Selector/4 -> Terminator10/1  "<T_GL_PNT_ATM_K>"
  Bus Creator2/1 -> ATM_DTTH/1  "ATM_DTTH"
  Bus Creator1/1 -> ATM_ELTH/1  "ATM_ELTH"
  ELTH_ATM/1 -> Bus Selector1/1
  Bus Selector1/1 -> Terminator2/1  "<PHI_RDTH_PNT_ATM_W>"
  Bus Selector1/2 -> Terminator3/1  "<PHI_MGTH_PNT_ATM_W>"
  Bus Selector1/3 -> Terminator4/1  "<PHI_INVTH_PNT_ATM_W>"
  BTTH_ATM/1 -> Bus Selector2/1
  Bus Selector2/2 -> Terminator9/1  "<PHI_BF_PNT_ATM_W>"
  Bus Selector2/1 -> Terminator8/1  "<PHI_BB_PNT_ATM_W>"
  Bus Creator3/1 -> ATM_BTTH/1  "ATM_BTTH"
  Signal Specification2/1 -> Bus Creator21/1  "T_ATM_PNT_Outside_degC"
  Bus Creator21/1 -> ATM_PNT_sensor/1  "ATM_PNT_sensor"
  DTTH_ATM/1 -> Bus Selector3/1
  Bus Selector3/1 -> Terminator/1  "<PHI_DFTH_PNT_ATM_W>"
  Bus Selector3/2 -> Terminator1/1  "<PHI_TMTH_PNT_ATM_W>"
  Environment/1 -> Bus Selector4/1
  Bus Selector4/2 -> Bus Creator/4  "<PHI_Environment_Sunlight_W>"
  Bus Selector4/1 -> degC->K/1(degC), Signal Specification2/1  "<ini_T_Environment_Outside_degC>"

== system EV_thermal_charger_2015a_jmaab/Vehicle/BAT_Hi_PNT ==
  I_CHG_PNT_A : Inport
  I_INV_PNT_DC_A : Inport  Port=2
  I_HVAC_PNT_A : Inport  Port=3
  T_BC_PNT_K : Inport  Port=4
  I_DCDC_PNT_Hi_A : Inport  Port=5
  Add : Sum  Inputs=++++
  BT_Hi_PNT : Subsystem
  Bus Creator9 : BusCreator  Inputs=2
  V_BT_Hi_PNT_V : Outport
  BT_Hi_PNT_sensor : Outport  Port=2
  PHI_BT_Hi_PNT_W : Outport  Port=3
  wires:
  BT_Hi_PNT/3(V_BT_Hi_PNT_V) -> V_BT_Hi_PNT_V/1
  BT_Hi_PNT/2(SOC_BT_Hi_PNT_per) -> Bus Creator9/2  "SOC_BT_Hi_PNT_per"
  BT_Hi_PNT/4(PHI_BT_Hi_PNT_W) -> PHI_BT_Hi_PNT_W/1
  BT_Hi_PNT/1(V_BT_Hi_PNT_V_1) -> Bus Creator9/1  "V_BT_Hi_PNT_V_1"
  Add/1 -> BT_Hi_PNT/1(I_BT_Hi_PNT_A)
  I_DCDC_PNT_Hi_A/1 -> Add/3
  Bus Creator9/1 -> BT_Hi_PNT_sensor/1  "BT_Hi_PNT_sensor"
  T_BC_PNT_K/1 -> BT_Hi_PNT/2(T_BC_PNT_K)
  I_CHG_PNT_A/1 -> Add/2
  I_INV_PNT_DC_A/1 -> Add/1
  I_HVAC_PNT_A/1 -> Add/4

== system EV_thermal_charger_2015a_jmaab/Vehicle/BK_PNT ==
  note: 制動力
  open_brake_BK_CNT_per1 : Inport
  "w_TR_PNT_radps " : Inport  Port=2
  Bus Selector15 : BusSelector  OutputSignals=open_brake_BK_CNT_per
  Constant2 : Constant  Value=tire_r
  Gain : Gain  Gain=-1
  Product6 : Product  RndMeth=Zero
  Q_cal3 : METI_Lib_vehicle_model/P_cal  Type_energy=回転運動  Type_output_energy=損失  Power_name=Pl_  t_Workspace_Name=BK_PNT_MECK_LOSS  P_VariableName=Pl_BK_PNT_MECK_LOSS  Across_VariableName=w_BK_PNT_MECK_LOSS  Throgh_VariableName=tq_BK_PNT_MECK_LOSS
  Terminator1 : Terminator
  Transfer Fcn : TransferFcn  Denominator=[BK_PNT_Tau_brake 1]
  per2F : Gain  Gain=BK_PNT_Pow_UL/100
  Trq_BK_PNT_Nm : Outport
  tag scope: tScope_MECK_Brk=global
  wires:
  Q_cal3/1 -> Terminator1/1
  Transfer Fcn/1 -> Product6/2
  Constant2/1 -> Product6/1
  Product6/1 -> Gain/1, Q_cal3/2
  "w_TR_PNT_radps "/1 -> Q_cal3/1
  Gain/1 -> Trq_BK_PNT_Nm/1  "trq_BK_PNT_Nm"
  per2F/1 -> Transfer Fcn/1
  open_brake_BK_CNT_per1/1 -> Bus Selector15/1
  Bus Selector15/1 -> [tScope_MECK_Brk], per2F/1  "<open_brake_BK_CNT_per>"

== system EV_thermal_charger_2015a_jmaab/Vehicle/BTTH ==
  BTTH_CNT_out : Inport
  PHI_BT_Hi_PNT_W : Inport  Port=2
  V_BT_Lo_PNT_V : Inport  Port=3
  Environment : Inport  Port=4
  ATM_BTTH : Inport  Port=5
  BTTH_PNT : Subsystem
  Bus Creator : BusCreator  Inputs=2
  Bus Creator4 : BusCreator  Inputs=1
  Bus Selector1 : BusSelector  OutputSignals=tgt_P_BTTH_CNT_BTHeater_W,V_BTTH_CNT_BTFan_V
  Bus Selector2 : BusSelector  OutputSignals=T_ATM_PNT_BB_K,T_ATM_PNT_BF_K
  Bus Selector4 : BusSelector  OutputSignals=ini_T_Environment_Outside_degC
  BTTH_sensor : Outport
  BTTH_ATM : Outport  Port=2
  T_BC_PNT_K : Outport  Port=3
  I_BTTH_PNT_A : Outport  Port=4
  wires:
  V_BT_Lo_PNT_V/1 -> BTTH_PNT/3(V_BT_Lo_PNT_V)
  BTTH_PNT/4(T_BC_PNT_degC) -> Bus Creator4/1  "T_BC_PNT_degC"
  BTTH_PNT/3(PHI_BF_PNT_ATM_W) -> Bus Creator/2
  BTTH_PNT/5(T_BC_PNT_K) -> T_BC_PNT_K/1
  BTTH_PNT/1(I_BTTH_PNT_A) -> I_BTTH_PNT_A/1
  PHI_BT_Hi_PNT_W/1 -> BTTH_PNT/4(PHI_BT_HI_PNT_W)
  Bus Creator4/1 -> BTTH_sensor/1  "BTTH_sensor"
  BTTH_CNT_out/1 -> Bus Selector1/1
  Bus Selector1/1 -> BTTH_PNT/1(tgt_P_BTTH_CNT_BTHeater_W)  "<tgt_P_BTTH_CNT_BTHeater_W>"
  Bus Selector1/2 -> BTTH_PNT/2(V_BTTH_CNT_BTFan_V)  "<V_BTTH_CNT_BTFan_V>"
  BTTH_PNT/2(PHI_BB_PNT_ATM_W) -> Bus Creator/1
  Bus Creator/1 -> BTTH_ATM/1  "BTTH_ATM"
  ATM_BTTH/1 -> Bus Selector2/1
  Bus Selector2/2 -> BTTH_PNT/6(T_ATM_PNT_BF_K)  "<T_ATM_PNT_BF_K>"
  Bus Selector2/1 -> BTTH_PNT/5(T_ATM_PNT_BB_K)  "<T_ATM_PNT_BB_K>"
  Environment/1 -> Bus Selector4/1
  Bus Selector4/1 -> BTTH_PNT/7(<ini_T_Environment_Outside_degC>)  "<ini_T_Environment_Outside_degC>"

== system EV_thermal_charger_2015a_jmaab/Vehicle/BT_Lo_PNT ==
  I_DCDC_PNT_Lo_A : Inport
  I_SH_PNT_A : Inport  Port=2
  I_BTTH_PNT_A : Inport  Port=3
  I_EL_PNT_A : Inport  Port=4
  Add4 : Sum  Inputs=++++
  BT_Lo_PNT : Subsystem
  V_BT_Lo_PNT_V : Outport
  wires:
  I_SH_PNT_A/1 -> Add4/1
  Add4/1 -> BT_Lo_PNT/1(I_BT_Lo_PNT_A)
  I_BTTH_PNT_A/1 -> Add4/3
  BT_Lo_PNT/1("V_BT_Lo_PNT_V ") -> V_BT_Lo_PNT_V/1
  I_EL_PNT_A/1 -> Add4/4
  I_DCDC_PNT_Lo_A/1 -> Add4/2

== system EV_thermal_charger_2015a_jmaab/Vehicle/CATH ==
  Heat_Resi_ELTH_PNT_AirconCore_KpW : Inport
  CATH_CNT_out : Inport  Port=2
  Environment : Inport  Port=3
  T_PTTH_PNT_CATH_K : Inport  Port=4
  V_BT_Hi_PNT_V : Inport  Port=5
  V_BT_Lo_PNT_V : Inport  Port=6
  v_VL_PNT_mps : Inport  Port=7
  ATM_CATH : Inport  Port=8
  Bus Creator : BusCreator  Inputs=4
  Bus Creator13 : BusCreator  Inputs=6
  Bus Selector1 : BusSelector  OutputSignals=T_ATM_PNT_GL_K,PHI_Environment_Sunlight_W,T_ATM_PNT_WA_K,T_ATM_PNT_AC_K
  Bus Selector4 : BusSelector  OutputSignals=ini_T_Environment_Outside_degC,add_T_Environment_CATH_degC
  Bus Selector7 : BusSelector  OutputSignals=P_CATH_CNT_Heatpomp_W,P_CATH_CNT_PTC_Heater_W,V_CATH_CNT_Aircon_Fan_V,P_CATH_CNT_SeatHT_W,req_V_CATH_CNT_RDFan_V
  CATH_PNT : Subsystem
  T_CATH_sensor : Outport
  PHI_CATH_PNT_PTTH_W : Outport  Port=2
  CATH_ATM : Outport  Port=3
  I_HVAC_PNT_A : Outport  Port=4
  I_SH_PNT_A : Outport  Port=5
  wires:
  Bus Selector7/3 -> CATH_PNT/8(V_CATH_CNT_Aircon_Fan_V)  "<V_CATH_CNT_Aircon_Fan_V>"
  T_PTTH_PNT_CATH_K/1 -> CATH_PNT/2(T_PTTH_PNT_CATH_K)
  Bus Selector7/1 -> CATH_PNT/6(P_CATH_CNT_Heatpomp_W)  "<P_CATH_CNT_Heatpomp_W>"
  CATH_PNT/5(T_PTC_PNT_degC) -> Bus Creator13/4  "T_PTC_PNT_degC"
  Bus Selector7/4 -> CATH_PNT/9(P_CATH_CNT_SeatHT_W)  "<P_CATH_CNT_SeatHT_W>"
  v_VL_PNT_mps/1 -> CATH_PNT/4(v_VL_PNT_kmph)
  Bus Selector7/2 -> CATH_PNT/7(P_CATH_CNT_PTC_Heater_W)  "<P_CATH_CNT_PTC_Heater_W>"
  Bus Creator13/1 -> T_CATH_sensor/1  "CATH_sensor"
  CATH_PNT/2(P_HVAC_PNT_W) -> Bus Creator13/1  "P_HVAC_PNT_W"
  V_BT_Hi_PNT_V/1 -> CATH_PNT/5(V_BT_Hi_PNT_V)
  CATH_PNT/3(T_AC_PNT_Outdoor_degC) -> Bus Creator13/2  "T_AC_PNT_Outdoor_degC"
  CATH_PNT/6(T_CABA_PNT_degC) -> Bus Creator13/5  "T_CABA_PNT_degC"
  CATH_PNT/7(T_SH_PNT_degC) -> Bus Creator13/6  "T_SH_PNT_degC"
  Bus Selector7/5 -> CATH_PNT/10(req_V_ELTH_CNT_RDFan_V)  "<req_V_CATH_CNT_RDFan_V>"
  CATH_PNT/4(T_AC_PNT_Indoor_degC) -> Bus Creator13/3  "T_AC_PNT_Indoor_degC"
  CATH_PNT/8(PHI_GL_PNT_ATM_W) -> Bus Creator/1
  Heat_Resi_ELTH_PNT_AirconCore_KpW/1 -> CATH_PNT/3(Heat_Resi_ELTH_PNT_AirconCore_KpW)
  V_BT_Lo_PNT_V/1 -> CATH_PNT/11(V_BT_Lo_PNT_V)
  CATH_PNT/9(PHI_WA_PNT_ATM_W) -> Bus Creator/2
  CATH_PNT/11(T_GL_PNT_ATM_K) -> Bus Creator/4
  CATH_PNT/13(I_SH_PNT_A) -> I_SH_PNT_A/1
  CATH_PNT/10(PHI_AC_PNT_ATM_W) -> Bus Creator/3
  CATH_PNT/1(PHI_CATH_PNT_PTTH_W) -> PHI_CATH_PNT_PTTH_W/1
  CATH_PNT/12(I_HVAC_PNT_A) -> I_HVAC_PNT_A/1
  CATH_CNT_out/1 -> Bus Selector7/1
  ATM_CATH/1 -> Bus Selector1/1
  Bus Selector1/1 -> CATH_PNT/1(T_ATM_PNT_GL_K)  "<T_ATM_PNT_GL_K>"
  Bus Selector1/2 -> CATH_PNT/12(PHI_ATM_PNT_Sunlight_W)  "<PHI_Environment_Sunlight_W>"
  Bus Selector1/4 -> CATH_PNT/14(T_ATM_PNT_AC_K)  "<T_ATM_PNT_AC_K>"
  Bus Selector1/3 -> CATH_PNT/13(T_ATM_PNT_WA_K)  "<T_ATM_PNT_WA_K>"
  Bus Creator/1 -> CATH_ATM/1  "CATH_ATM"
  Environment/1 -> Bus Selector4/1
  Bus Selector4/1 -> CATH_PNT/15(ini_T_Environment_Outside_degC)  "<ini_T_Environment_Outside_degC>"
  Bus Selector4/2 -> CATH_PNT/16(<add_T_Environment_CATH_degC>)  "<add_T_Environment_CATH_degC>"

== system EV_thermal_charger_2015a_jmaab/Vehicle/CHG_PNT ==
  note: CHG_PNT
  CHG_CNT_out : Inport
  V_CHG_PNT_V : Inport  Port=2
  Bus Creator23 : BusCreator  Inputs=1
  Bus Selector : BusSelector  OutputSignals=tgt_I_CHG_CNT_Charge_A
  Signal Specification : SignalSpecification
  Signal Specification1 : SignalSpecification
  Terminator : Terminator
  CHG_PNT_sensor : Outport
  I_CHG_PNT_A : Outport  Port=2
  wires:
  V_CHG_PNT_V/1 -> Signal Specification1/1, Terminator/1
  Bus Creator23/1 -> CHG_PNT_sensor/1  "CHG_PNT_sensor"
  Signal Specification/1 -> I_CHG_PNT_A/1  "I_CHG_PNT_A"
  Bus Selector/1 -> Signal Specification/1  "<tgt_I_CHG_CNT_Charge_A>"
  CHG_CNT_out/1 -> Bus Selector/1
  Signal Specification1/1 -> Bus Creator23/1  "V_CHG_PNT_V"

== system EV_thermal_charger_2015a_jmaab/Vehicle/CNT ==
  VL_sensor : Inport
  Driver_Input : Inport  Port=2
  BK_CNT : Subsystem
  BTTH_CNT : Subsystem
  Bus Creator18 : BusCreator  Inputs=6
  Bus Selector1 : BusSelector  OutputSignals=VL_PNT_sensor,DCDC_PNT_sensor,MG_sensor,INV_sensor,ELTH_sensor,CATH_sensor,ATM_PNT_sensor,BTTH_sensor,CHG_PNT_sensor,BT_Hi_PNT_sensor
  CATH_CNT : Subsystem
  CHG_CNT : Subsystem
  EL_TH_CNT : Subsystem
  MG_CNT : Subsystem
  VCU_CNT : Subsystem
  CNT_out : Outport
  wires:
  Driver_Input/1 -> [Driver_input], VCU_CNT/1(Driver_Input)
  VL_sensor/1 -> Bus Selector1/1
  Bus Creator18/1 -> CNT_out/1  "CNT_out"
  BK_CNT/1(BK_CNT_out) -> Bus Creator18/1
  MG_CNT/1(MG_CNT_out) -> Bus Creator18/2
  EL_TH_CNT/1(EL_TH_CNT_out) -> Bus Creator18/3
  CATH_CNT/2(CATH_CNT_out) -> Bus Creator18/4
  BTTH_CNT/1(BTTH_CNT_out) -> Bus Creator18/5
  CHG_CNT/1(CHG_CNT_out) -> Bus Creator18/6
  Bus Selector1/3 -> VCU_CNT/4(MG_sensor), MG_CNT/2(MG_sensor)  "<MG_sensor>"
  Bus Selector1/4 -> MG_CNT/3(INV_sensor)  "<INV_sensor>"
  Bus Selector1/5 -> EL_TH_CNT/1(PTTH_sensor)  "<ELTH_sensor>"
  Bus Selector1/6 -> VCU_CNT/5(CATH_sensor), CATH_CNT/1(CATH_sensor)  "<CATH_sensor>"
  Bus Selector1/8 -> BTTH_CNT/1(BTTH_sensor)  "<BTTH_sensor>"
  Bus Selector1/7 -> CATH_CNT/2(ATM_PNT_sensor)  "<ATM_PNT_sensor>"
  Bus Selector1/9 -> CHG_CNT/2(CHG_PNT_sensor)  "<CHG_PNT_sensor>"
  Bus Selector1/10 -> VCU_CNT/6(BT_Hi_PNT_sensor), CHG_CNT/3(BT_Hi_PNT_sensor)  "<BT_Hi_PNT_sensor>"
  Bus Selector1/2 -> VCU_CNT/3(DCDC_PNT_sensor)  "<DCDC_PNT_sensor>"
  Bus Selector1/1 -> VCU_CNT/2(VL_sensor), CATH_CNT/3(VL_sensor)  "<VL_PNT_sensor>"
  [Driver_input] -> BK_CNT/2(DriverDmnd)
  [Driver_input] -> CATH_CNT/4(Driver_Input)
  [Driver_input] -> CHG_CNT/1(DriverDmnd)
  VCU_CNT/1(VCU_CNT_CAN_Tx) -> MG_CNT/1(VCU_CNT_CAN_Tx), BK_CNT/1(VCU_CNT_CAN_Tx)
  CATH_CNT/1(CATH_CNT_CAN_Tx) -> EL_TH_CNT/2(CATH_CNT_CAN_Tx)

== system EV_thermal_charger_2015a_jmaab/Vehicle/DCDC_PNT ==
  V_BT_Hi_PNT_V : Inport
  V_BT_Lo_PNT_V : Inport  Port=2
  Bus Creator19 : BusCreator  Inputs=1
  DCDC_PNT : Subsystem
  DCDC_PNT_sensor : Outport
  I_DCDC_PNT_Lo_A : Outport  Port=2
  I_DCDC_PNT_Hi_A : Outport  Port=3
  wires:
  DCDC_PNT/2(I_DCDC_PNT_Hi_A) -> I_DCDC_PNT_Hi_A/1
  DCDC_PNT/1(P_DCDC_PNT_W) -> Bus Creator19/1  "P_DCDC_PNT_W"
  Bus Creator19/1 -> DCDC_PNT_sensor/1  "DCDC_PNT_sensor"
  DCDC_PNT/3(I_DCDC_PNT_Lo_A) -> I_DCDC_PNT_Lo_A/1
  V_BT_Lo_PNT_V/1 -> DCDC_PNT/2(V_BT_Lo_PNT_V)
  V_BT_Hi_PNT_V/1 -> DCDC_PNT/1(V_BT_Hi_PNT_V)

== system EV_thermal_charger_2015a_jmaab/Vehicle/DTTH ==
  PHI_DT_PNT : Inport
  PHI_MGTH_PNT_PTTH_W : Inport  Port=2
  Environment : Inport  Port=3
  PHI_CATH_PNT_PTTH_W : Inport  Port=4
  ATM_DTTH : Inport  Port=5
  Bus Creator : BusCreator  Inputs=2
  Bus Creator1 : BusCreator  Inputs=2
  Bus Creator24 : BusCreator  Inputs=1
  Bus Selector : BusSelector  OutputSignals=PHI_DF_PNT_W,PHI_TM_PNT_W
  Bus Selector4 : BusSelector  OutputSignals=ini_T_Environment_Outside_degC,add_T_Environment_PTTH_ELTH_degC
  DTTH_PNT : Subsystem
  T_DTTH : Outport
  DTTH_sensor : Outport  Port=2
  DTTH_ATM : Outport  Port=3
  T_PTTH_PNT_CATH_K : Outport  Port=4
  T_TMTH_PNT_ELTH_K : Outport  Port=5
  wires:
  DTTH_PNT/4("PHI_DFTH_PNT_ATM_W ") -> Bus Creator1/1
  ATM_DTTH/1 -> DTTH_PNT/5(ATM_DTTH)
  DTTH_PNT/5("PHI_TMTH_PNT_ATM_W ") -> Bus Creator1/2
  PHI_MGTH_PNT_PTTH_W/1 -> DTTH_PNT/4(PHI_MGTH_PNT_PTTH_W)
  DTTH_PNT/6(T_TMTH_PNT_TF_degC) -> Bus Creator24/1  "T_TMTH_PNT_TF_degC"
  DTTH_PNT/2(T_DFTH_PNT_TM_K) -> Bus Creator/2
  DTTH_PNT/1(T_TMTH_PNT_TM_K) -> Bus Creator/1
  DTTH_PNT/7(T_PTTH_PNT_CATH_K) -> T_PTTH_PNT_CATH_K/1
  Bus Creator24/1 -> DTTH_sensor/1  "DTTH_sensor"
  DTTH_PNT/3(T_TMTH_PNT_ELTH_K) -> T_TMTH_PNT_ELTH_K/1
  PHI_CATH_PNT_PTTH_W/1 -> DTTH_PNT/3("PHI_CATH_PNT_PTTH_W ")
  Bus Creator/1 -> T_DTTH/1  "T_DTTH"
  PHI_DT_PNT/1 -> Bus Selector/1
  Bus Selector/1 -> DTTH_PNT/1(PHI_DF_PNT_W)  "<PHI_DF_PNT_W>"
  Bus Selector/2 -> DTTH_PNT/2(PHI_TM_PNT_W)  "<PHI_TM_PNT_W>"
  Bus Creator1/1 -> DTTH_ATM/1  "DTTH_ATM"
  Bus Selector4/1 -> DTTH_PNT/6(<ini_T_Environment_Outside_degC>)  "<ini_T_Environment_Outside_degC>"
  Environment/1 -> Bus Selector4/1
  Bus Selector4/2 -> DTTH_PNT/7(<add_T_Environment_PTTH_ELTH_degC>)  "<add_T_Environment_PTTH_ELTH_degC>"

== system EV_thermal_charger_2015a_jmaab/Vehicle/DT_PNT ==
  Trq_MG_PNT_Nm : Inport
  T_DTTH : Inport  Port=2
  w_TR_PNT_radps : Inport  Port=3
  Bus Creator : BusCreator  Inputs=2
  Bus Selector : BusSelector  OutputSignals=T_TMTH_PNT_TM_K,T_DFTH_PNT_TM_K
  DF_PNT : Subsystem
      mask Display: image(imread('picture\回転変換.png'))
  TM_PNT : Subsystem
      mask Display: image(imread('パワトレ　AT.jpg'))
  Trq_DF_PNT_DN_Nm : Outport
  PHI_DT_PNT : Outport  Port=2
  w_TM_PNT_UP_radps : Outport  Port=3
  wires:
  DF_PNT/2(Trq_DF_PNT_DN_Nm) -> Trq_DF_PNT_DN_Nm/1
  DF_PNT/3("PHI_DF_PNT_W ") -> Bus Creator/1
  DF_PNT/1(Trq_DF_PNT_UP_Nm) -> TM_PNT/1(Trq_DF_PNT_UP_Nm)
  TM_PNT/3(w_TM_PNT_UP_radps) -> w_TM_PNT_UP_radps/1
  TM_PNT/1("w_TM_PNT_DN_radps ") -> DF_PNT/2(w_TM_PNT_DN_radps)
  w_TR_PNT_radps/1 -> DF_PNT/1("ｗ_TR_PNT_radps ")
  Bus Selector/2 -> DF_PNT/3("T_DFTH_PNT_TM_K ")  "<T_DFTH_PNT_TM_K>"
  Trq_MG_PNT_Nm/1 -> TM_PNT/2("Trq_MG_PNT_Nm ")
  TM_PNT/2(PHI_TM_PNT_W) -> Bus Creator/2
  Bus Creator/1 -> PHI_DT_PNT/1  "PHI_DT_PNT"
  T_DTTH/1 -> Bus Selector/1
  Bus Selector/1 -> TM_PNT/3(T_TMTH_PNT_TM_K)  "<T_TMTH_PNT_TM_K>"

== system EV_thermal_charger_2015a_jmaab/Vehicle/ELTH ==
  PHI_MG_PNT_W : Inport
  PHI_INV_PNT_W : Inport  Port=2
  Environment : Inport  Port=3
  EL_TH_CNT_out : Inport  Port=4
  v_VL_PNT_mps : Inport  Port=5
  T_TMTH_PNT_ELTH_K : Inport  Port=6
  ATM_ELTH : Inport  Port=7
  Bus Creator1 : BusCreator  Inputs=3
  Bus Creator14 : BusCreator  Inputs=3
  Bus Selector1 : BusSelector  OutputSignals=T_ATM_PNT_RD_K,T_ATM_PNT_MG_K,T_ATM_PNT_INV_K
  Bus Selector4 : BusSelector  OutputSignals=ini_T_Environment_Outside_degC,add_T_Environment_PTTH_ELTH_degC
  Bus Selector9 : BusSelector  OutputSignals=req_V_ELTH_CNT_RDFan_V,V_ELTH_CNT_WP_V
  ELTH_PNT : Subsystem
  T_INVTH_PNT_K : Outport
  T_MGTH_PNT_K : Outport  Port=2
  ELTH_sensor : Outport  Port=3
  PHI_MGTH_PNT_PTTH_W : Outport  Port=4
  ELTH_ATM : Outport  Port=5
  Heat_Resi_ELTH_PNT_AirconCore_KpW : Outport  Port=6
  wires:
  Bus Selector9/2 -> ELTH_PNT/6(V_ELTH_CNT_WP_V)  "<V_ELTH_CNT_WP_V>"
  Bus Creator14/1 -> ELTH_sensor/1  "ELTH_sensor"
  ELTH_PNT/5("PHI_RDTH_PNT_ATM_W ") -> Bus Creator1/2
  Bus Selector9/1 -> ELTH_PNT/5(V_ELTH_CNT_RDFan_V)  "<req_V_ELTH_CNT_RDFan_V>"
  ELTH_PNT/4("PHI_MGTH_PNT_ATM_W ") -> Bus Creator1/1
  ELTH_PNT/2(T_MGTH_PNT_MGHousing_degC) -> Bus Creator14/2  "T_MGTH_PNT_MGHousing_degC"
  ELTH_PNT/3(T_INVTH_PNT_INVHeatsink_degC) -> Bus Creator14/3  "T_INVTH_PNT_INVHeatsink_degC"
  T_TMTH_PNT_ELTH_K/1 -> ELTH_PNT/8(T_TMTH_PNT_ELTH_K)
  ELTH_PNT/7(Heat_Resi_ELTH_PNT_AirconCore_KpW) -> Heat_Resi_ELTH_PNT_AirconCore_KpW/1  "Heat_Resi_ELTH_PNT_AirconCore_KpW"
  ELTH_PNT/1(T_RDTH_PNT_RDCoolant_degC) -> Bus Creator14/1  "T_RDTH_PNT_RDCoolant_degC"
  ELTH_PNT/8(T_INVTH_PNT_K) -> T_INVTH_PNT_K/1
  PHI_INV_PNT_W/1 -> ELTH_PNT/7(PHI_INV_PNT_W)
  ELTH_PNT/6("PHI_INVTH_PNT_ATM_W ") -> Bus Creator1/3
  ELTH_PNT/9(T_MGTH_PNT_K) -> T_MGTH_PNT_K/1
  PHI_MG_PNT_W/1 -> ELTH_PNT/4(PHI_MG_PNT_W)
  ELTH_PNT/10(PHI_MGTH_PNT_PTTH_W) -> PHI_MGTH_PNT_PTTH_W/1
  v_VL_PNT_mps/1 -> ELTH_PNT/3(v_VL_PNT_mps)
  EL_TH_CNT_out/1 -> Bus Selector9/1
  ATM_ELTH/1 -> Bus Selector1/1
  Bus Selector1/1 -> ELTH_PNT/1(T_ATM_PNT_RD_K)  "<T_ATM_PNT_RD_K>"
  Bus Selector1/2 -> ELTH_PNT/2(T_ATM_PNT_MG_K)  "<T_ATM_PNT_MG_K>"
  Bus Selector1/3 -> ELTH_PNT/9(T_ATM_PNT_INV_K)  "<T_ATM_PNT_INV_K>"
  Bus Creator1/1 -> ELTH_ATM/1  "ELTH_ATM"
  Environment/1 -> Bus Selector4/1
  Bus Selector4/1 -> ELTH_PNT/10(In10)  "<ini_T_Environment_Outside_degC>"
  Bus Selector4/2 -> ELTH_PNT/11(In11)  "<add_T_Environment_PTTH_ELTH_degC>"
